simulink model "VTOL_6D0F_control"  (R2023a)
settings: Solver=VariableStepAuto  StartTime=0.0  StopTime=100  RelTol=1e-3
values from neighbouring files (symbols this model uses):
  A_lat = [Y_beta/u0  Y_p/u0  -(1-(Y_r)/(u0))  g/u0 ; L_beta  L_p  L_r  0  ;N_beta  N_p N_r 0  ; 0 1 0 0 ]    [vtol_script.m]
  A_long = [Xu Xw   0  -g  0; Zu Zw  u0 0  0 ; Mu+Mwdot*Zu  Mw+Mwdot*Zw  Mq+Mwdot*u0  0  0; 0  0  1  0  0 ; 0 0 0 k0  0]    [vtol_script.m]
  B_lat = [0 Y_delr/u0 ; L_dela   L_delr; N_dela N_delr ; 0 0]    [vtol_script.m]
  B_long = [ Xd XdT ; Zde   ZdT; Md  MdT; 0 0 ;0 0]    [vtol_script.m]
  C_lat = eye(4)    [vtol_script.m]
  C_long = eye(5)    [vtol_script.m]
  C_p = K_T/(0.5*rho*S_p*(R_p)^2)    (= 0.0365795108738)    [vtol_script.m]
  D_lat = zeros(4,2)    [vtol_script.m]
  D_long = [ 0 0; 0 0; 0 0; 0 0; 0 0]    [vtol_script.m]
  guidance_mode_on = 1    [vtol_script.m]
  K_motor = 942.3726    [vtol_script.m]
  q_motor = 283    [vtol_script.m]
  R_p = 0.3556/2    (= 0.1778)    [vtol_script.m]
  S_p = pi*(R_p)^2    (= 0.0993146659031)    [vtol_script.m]
  u0 = 16    [vtol_script.m]
libraries: simulink_extras x26, slpidlib x6, aerolibatmos2 x1
settings Model: Creator=manup  LastModifiedBy=manup

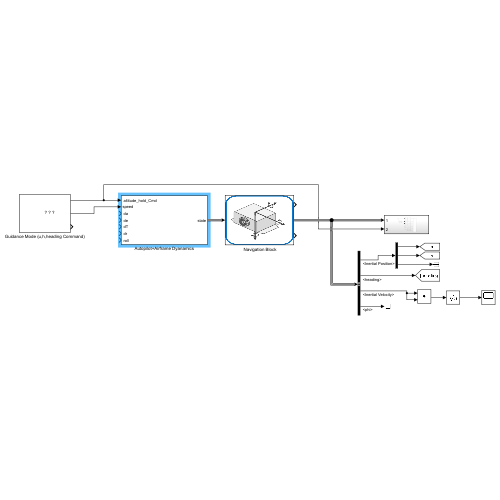
[thumbnail: Simulink's stored preview of the top-level diagram]
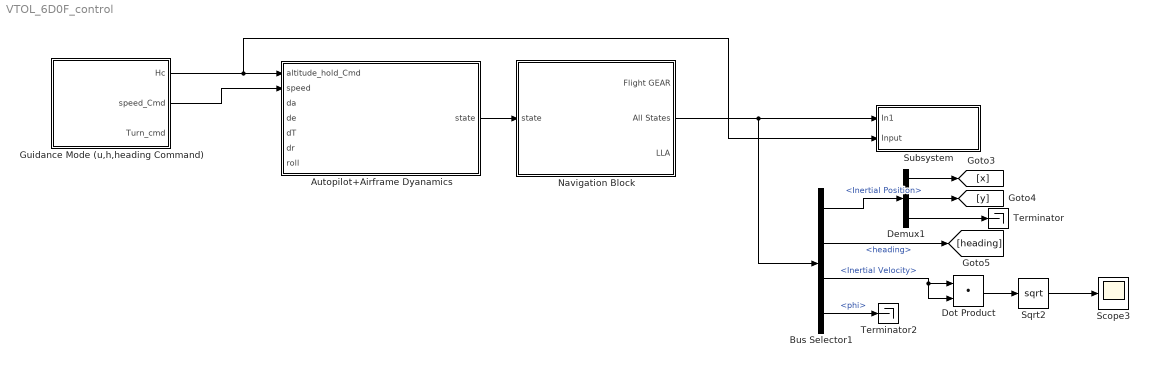
== system VTOL_6D0F_control ==
  " Navigation Block" : Subsystem
      mask Display: image('sensor.png'); % Use "Edit Image" on toolstrip to change.
  Autopilot+Airframe Dyanamics : Subsystem
  Bus Selector1 : BusSelector  OutputSignals=Inertial Position,heading,Inertial Velocity,states.phi
  Demux1 : Demux  Outputs=03
  Dot Product : DotProduct  OutDataTypeStr=Inherit: Inherit via internal rule
  Guidance Mode (u,h,heading Command) : Subsystem
      mask Display: image('guidance.jpg'); % Use "Edit Image" on toolstrip to change.
  Scope3 : Scope
  Sqrt2 : Sqrt
  Subsystem : Subsystem
  Terminator : Terminator
  Terminator2 : Terminator
  wires:
  " Navigation Block"/2(" All States") -> Bus Selector1/1, Subsystem/1(In1)
  Demux1/1 -> [x]
  Bus Selector1/4 -> Terminator2/1  "<phi>"
  Autopilot+Airframe Dyanamics/1(" state") -> " Navigation Block"/1(" state")
  Demux1/3 -> Terminator/1
  Demux1/2 -> [y]
  Bus Selector1/2 -> [heading]  "<heading>"
  Bus Selector1/3 -> Dot Product/2, Dot Product/1  "<Inertial Velocity>"
  Guidance Mode (u,h,heading Command)/1(Hc) -> Autopilot+Airframe Dyanamics/1(" altitude_hold_Cmd"), Subsystem/2(Input)
  Dot Product/1 -> Sqrt2/1
  Guidance Mode (u,h,heading Command)/2(speed_Cmd) -> Autopilot+Airframe Dyanamics/2(speed)
  Bus Selector1/1 -> Demux1/1  "<Inertial Position>"
  Sqrt2/1 -> Scope3/1

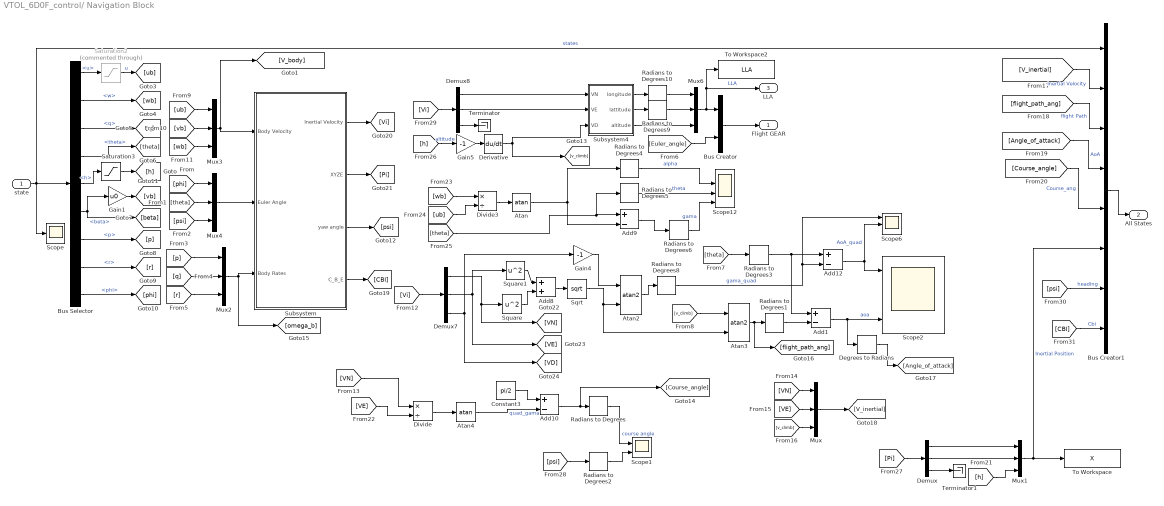
== system VTOL_6D0F_control/ Navigation Block ==
  " state" : Inport
  Add{1,9..10,12} (4 alike) : Sum  Inputs=+-
  Add8 : Sum
  Atan : Trigonometry  Operator=atan
  Atan2 : Trigonometry  Operator=atan2
  Atan3 : Trigonometry  Operator=atan2
  Atan4 : Trigonometry  Operator=atan
  Bus Creator : BusCreator  Inputs=2
  Bus Creator1 : BusCreator  Inputs=8
  Bus Selector : BusSelector  OutputSignals=u,w,q,theta,h,beta,p,r,phi
  Constant3 : Constant  Value=pi/2
  Degrees to Radians : simulink_extras/Transformations/Degrees to Radians
  Demux : Demux  Outputs=03
  Demux7 : Demux  Outputs=03
  Demux8 : Demux  Outputs=03
  Derivative : Derivative
  Divide : Product  Inputs=*/
  Divide3 : Product  Inputs=*/
  Gain1 : Gain  Gain=u0
  Gain4 : Gain  Gain=-1
  Gain5 : Gain  Gain=-1
  Mux{,1..4,6} (6 alike) : Mux  Inputs=03
  Radians to Degrees{,1..6,8..10} (10 alike) : simulink_extras/Transformations/Radians to Degrees
  Saturation2 : Saturate  Commented=through  UpperLimit=20  LowerLimit=0
  Saturation3 : Saturate  UpperLimit=0  LowerLimit=-6000
  Scope : Scope
  Scope1 : Scope  NumInputPorts=2
  Scope12 : Scope  NumInputPorts=4
  Scope2 : Scope  NumInputPorts=3
  Scope6 : Scope  NumInputPorts=3
  Sqrt : Sqrt
  Square : Math  Operator=square
  Square1 : Math  Operator=square
  Subsystem : Subsystem
  Subsystem4 : Subsystem
  Terminator : Terminator
  Terminator1 : Terminator
  To Workspace : ToWorkspace  VariableName=X  SampleTime=-1
  To Workspace2 : ToWorkspace  VariableName=LLA  SampleTime=-1
  " Flight GEAR" : Outport
  " All States" : Outport  Port=2
  LLA : Outport  Port=3
  wires:
  " state"/1 -> Bus Creator1/1, Bus Selector/1, Scope/1  "states"
  Saturation3/1 -> [h]
  Gain1/1 -> [vb]
  Saturation2/1 -> [ub]  "u"
  Bus Selector/1 -> Saturation2/1  "<u>"
  Bus Selector/3 -> [q]  "<q>"
  Bus Selector/6 -> Gain1/1, [beta]  "<beta>"
  Bus Selector/8 -> [r]  "<r>"
  Bus Selector/4 -> [theta]  "<theta>"
  Bus Selector/5 -> Saturation3/1  "<h>"
  Bus Selector/9 -> [phi]  "<phi>"
  Bus Selector/7 -> [p]  "<p>"
  Bus Selector/2 -> [wb]  "<w>"
  Radians to Degrees4/1 -> Scope12/2  "alpha"
  Demux7/1 -> [VN], Square/1
  Radians to Degrees6/1 -> Scope12/4  "gama"
  Demux7/3 -> [VD], Gain4/1
  [wb] -> Divide3/1
  Gain4/1 -> Atan2/1
  Add12/1 -> Scope2/1, Scope6/2  "AoA_quad"
  [theta] -> Add9/1, Radians to Degrees5/1
  [ub] -> Divide3/2
  [h] -> Gain5/1  "altitude"
  Atan4/1 -> Add10/2  "quad_gama"
  Add10/1 -> [Course_angle], Radians to Degrees/1
  Gain5/1 -> Derivative/1
  Atan2/1 -> Radians to Degrees8/1
  Add8/1 -> Sqrt/1
  [Vi] -> Demux7/1
  Radians to Degrees5/1 -> Scope12/3  "theta"
  Divide3/1 -> Atan/1
  Constant3/1 -> Add10/1
  Add9/1 -> Radians to Degrees6/1
  Atan/1 -> Radians to Degrees4/1, Add9/2
  Square/1 -> Add8/2
  Square1/1 -> Add8/1
  Radians to Degrees8/1 -> Scope6/1, Add12/2  "gama_quad"
  [VN] -> Divide/1
  Demux7/2 -> [VE], Square1/1
  [VE] -> Divide/2
  Subsystem/1(" Inertial Velocity ") -> [Vi]
  Subsystem/2(XYZE) -> [Pi]
  Radians to Degrees/1 -> Scope1/1  "course angle"
  [ub] -> Mux3/1
  [vb] -> Mux3/2
  [wb] -> Mux3/3
  Mux3/1 -> [V_body], Subsystem/1(" Body Velocity")
  Mux6/1 -> LLA/1, To Workspace2/1, Bus Creator/1  "LLA"
  Radians to Degrees10/1 -> Mux6/1
  [Vi] -> Demux8/1
  Radians to Degrees9/1 -> Mux6/2
  Demux8/1 -> Subsystem4/1(" VN")
  Subsystem4/2(" lattitude") -> Radians to Degrees9/1
  Subsystem4/3(" altitude") -> Mux6/3
  Subsystem4/1(longitude) -> Radians to Degrees10/1
  Demux8/2 -> Subsystem4/2(" VE")
  Bus Creator/1 -> " Flight GEAR"/1
  Sqrt/1 -> Atan2/2, Atan3/2
  Derivative/1 -> Subsystem4/3(VD), [v_climb]
  Atan3/1 -> [flight_path_ang], Radians to Degrees1/1
  Radians to Degrees1/1 -> Add1/2
  Add1/1 -> Scope2/3, Degrees to Radians/1  "aoa"
  Mux4/1 -> Subsystem/2(" Euler Angle ")
  [phi] -> Mux4/1
  [theta] -> Mux4/2
  [psi] -> Mux4/3
  [p] -> Mux2/1
  [q] -> Mux2/2
  [r] -> Mux2/3
  Mux2/1 -> [omega_b], Subsystem/3(Body Rates)
  Demux8/3 -> Terminator/1
  Subsystem/3(yaw angle) -> [psi]
  [Euler_angle] -> Bus Creator/2
  [theta] -> Radians to Degrees3/1
  [v_climb] -> Atan3/1
  [VN] -> Mux/1
  [VE] -> Mux/2
  [v_climb] -> Mux/3
  Mux/1 -> [V_inertial]
  Bus Creator1/1 -> " All States"/1
  [V_inertial] -> Bus Creator1/2  "Inertial Velocity"
  [flight_path_ang] -> Bus Creator1/3  "flight Path"
  [Angle_of_attack] -> Bus Creator1/4  "AoA"
  [Course_angle] -> Bus Creator1/5  "Course_ang"
  Mux1/1 -> To Workspace/1, Bus Creator1/6  "Inertial Position"
  [h] -> Mux1/3
  [Pi] -> Demux/1
  Demux/1 -> Mux1/1
  Demux/2 -> Mux1/2
  Demux/3 -> Terminator1/1
  [psi] -> Radians to Degrees2/1
  Divide/1 -> Atan4/1
  Radians to Degrees2/1 -> Scope1/2
  [psi] -> Bus Creator1/7  "heading"
  Radians to Degrees3/1 -> Add1/1, Add12/1
  Degrees to Radians/1 -> [Angle_of_attack]
  Subsystem/4(C_B_E) -> [CBI]
  [CBI] -> Bus Creator1/8  "Cbi"

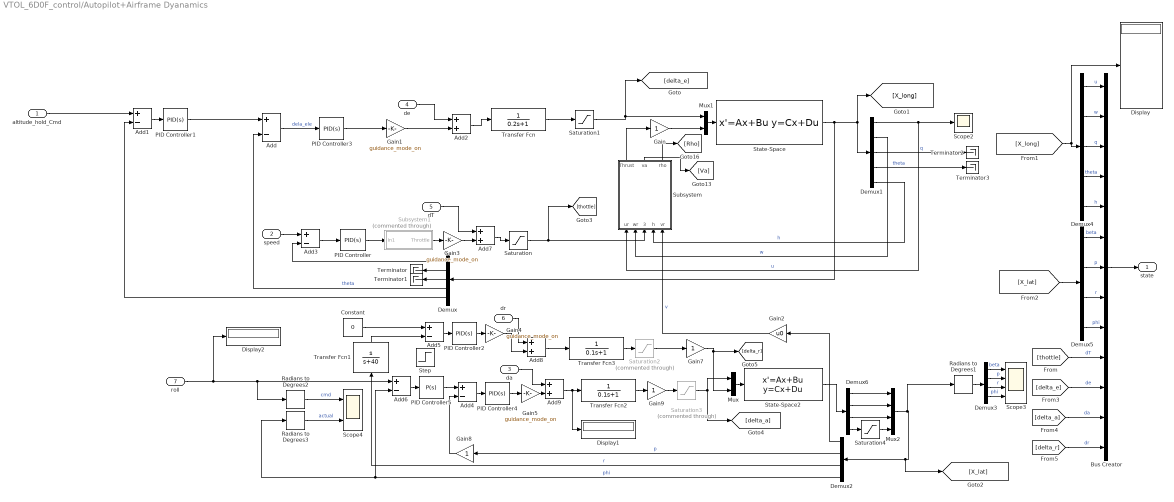
== system VTOL_6D0F_control/Autopilot+Airframe Dyanamics ==
  " altitude_hold_Cmd" : Inport
  speed : Inport  Port=2
  " da" : Inport  Port=3
  " de" : Inport  Port=4
  " dT" : Inport  Port=5
  " dr" : Inport  Port=6
  " roll" : Inport  Port=7
  Add{,1,3..6} (6 alike) : Sum  Inputs=+-
  Add{2,7..9} (4 alike) : Sum
  Bus Creator : BusCreator  Inputs=13
  Constant : Constant  Value=0
  Demux : Demux  Outputs=05
  Demux1 : Demux  Outputs=05
  Demux{2..3,5..6} (4 alike) : Demux  Outputs=04
  Demux4 : Demux  Outputs=05
  Display : Display
  Display1 : Display
  Display2 : Display
  Gain : Gain
  Gain{1,3..5} (4 alike) : Gain  Gain=guidance_mode_on
  Gain2 : Gain  Gain=u0
  Gain7 : Gain
  Gain8 : Gain  Gain=1
  Gain9 : Gain
  Mux : Mux  Inputs=2
  Mux1 : Mux  Inputs=2
  Mux2 : Mux  Inputs=04
  PID Controller : slpidlib/PID Controller  Controller=PID  Form=Parallel  TimeDomain=Continuous-time  UseExternalTs=off  SampleTime=-1  IntegratorMethod=Forward Euler  FilterMethod=Forward Euler  ControllerParametersSource=internal  P=2289.48575834425  I=747.437446989408  UseKiTs=off  D=-902.083389576885  N=0.350006005216069  UseFilter=on  TunerSelectOption=Transfer Function Based (PID Tuner App)  InitialConditionSource=internal  InitialConditionForIntegrator=0  InitialConditionForFilter=0  DifferentiatorICPrevScaledInput=0  ExternalReset=none  TrackingMode=off  Kt=1  LimitOutput=off  SatLimitsSource=internal  UpperSaturationLimit=inf  LowerSaturationLimit=-inf  LinearizeAsGain=on  AntiWindupMode=none  Kb=1  LimitIntegrator=off  UpperIntegratorSaturationLimit=inf  LowerIntegratorSaturationLimit=-inf  POutMin=[]  POutMax=[]  IOutMin=[]  IOutMax=[]  DOutMin=[]  DOutMax=[]  NOutMin=[]  NOutMax=[]  SumOutMin=[]  SumOutMax=[]  SaturationOutMin=[]  SaturationOutMax=[]  PParamMin=[]  PParamMax=[]  IParamMin=[]  IParamMax=[]  DParamMin=[]  DParamMax=[]  NParamMin=[]  NParamMax=[]  KbParamMin=[]  KbParamMax=[]  KtParamMin=[]  KtParamMax=[]  KbOutMin=[]  KbOutMax=[]  KtOutMin=[]  KtOutMax=[]  IntegratorOutMin=[]  IntegratorOutMax=[]  FilterOutMin=[]  FilterOutMax=[]  SumI1OutMin=[]  SumI1OutMax=[]  SumI2OutMin=[]  SumI2OutMax=[]  SumI3OutMin=[]  SumI3OutMax=[]  SumI4OutMin=[]  SumI4OutMax=[]  SumDOutMin=[]  SumDOutMax=[]  DifferentiatorOutMin=[]  DifferentiatorOutMax=[]  FilterDiffOutCoefMin=[]  FilterDiffOutCoefMax=[]  ReciprocalOutMin=[]  ReciprocalOutMax=[]  SumDenOutMin=[]  SumDenOutMax=[]  SumNumOutMin=[]  SumNumOutMax=[]  DivideOutMin=[]  DivideOutMax=[]  UdiffTsProdOutMin=[]  UdiffTsProdOutMax=[]  NTsProdOutMin=[]  NTsProdOutMax=[]  UintegralTsProdOutMin=[]  UintegralTsProdOutMax=[]  UngainTsProdOutMin=[]  UngainTsProdOutMax=[]  ClampingZeroOutDataTypeStr=Inherit: Inherit via back propagation  ClampingZeroOutMin=[]  ClampingZeroOutMax=[]  FilterDenConstantOutDataTypeStr=Inherit: Inherit via back propagation  FilterDenConstantOutMin=[]  FilterDenConstantOutMax=[]  PCopyOutDataTypeStr=Inherit: Inherit via back propagation  PCopyOutMin=[]  PCopyOutMax=[]  NCopyOutDataTypeStr=Inherit: Inherit via back propagation  NCopyOutMin=[]  NCopyOutMax=[]  IntegratorContinuousStateAttributes=''  IntegratorStateMustResolveToSignalObject=off  IntegratorRTWStateStorageClass=Auto  FilterContinuousStateAttributes=''  FilterStateMustResolveToSignalObject=off  FilterRTWStateStorageClass=Auto  ParallelPVariant=InternalParameters  IdealPVariant=Disabled  IVariant=InternalParameters  DVariant=InternalParameters  IntegratorVariant=Continuous  SatVariant=Disabled  AWVariant=Passthrough  PCopyVariant=Disabled  TRVariant=Disabled  FdbkBlocksVariant=Forward  IdealPFdbkVariant=Disabled  SatFdbkVariant=Disabled  DerivativeFilterVariant=ContFilter  NVariant=InternalParameters  NCopyVariant=Disabled  FilterICVariant=InternalICsFilter  IntegratorICVariant=InternalICs  ExternalResetVariant=Disabled  TRSumVariant=Passthrough  SumFdbkVariant=Disabled  SumVariant=Sum_PID  TsampFilterVariant=InternalTs  TsampNgainVariant=Passthrough  TsampIntegralVariant=Disabled_SignalSpec  ExternalSaturationOutDataTypeStr=Inherit: Same as second input
  PID Controller1 : slpidlib/PID Controller  Controller=PID  Form=Parallel  TimeDomain=Continuous-time  UseExternalTs=off  SampleTime=-1  IntegratorMethod=Forward Euler  FilterMethod=Forward Euler  ControllerParametersSource=internal  P=-0.00607559609713456  I=-7.12616824701196e-05  UseKiTs=off  D=-0.104565196845911  N=0.496463634396692  UseFilter=on  TunerSelectOption=Transfer Function Based (PID Tuner App)  InitialConditionSource=internal  InitialConditionForIntegrator=0  InitialConditionForFilter=0  DifferentiatorICPrevScaledInput=0  ExternalReset=none  TrackingMode=off  Kt=1  LimitOutput=off  SatLimitsSource=internal  UpperSaturationLimit=inf  LowerSaturationLimit=-inf  LinearizeAsGain=on  AntiWindupMode=none  Kb=1  LimitIntegrator=off  UpperIntegratorSaturationLimit=inf  LowerIntegratorSaturationLimit=-inf  POutMin=[]  POutMax=[]  IOutMin=[]  IOutMax=[]  DOutMin=[]  DOutMax=[]  NOutMin=[]  NOutMax=[]  SumOutMin=[]  SumOutMax=[]  SaturationOutMin=[]  SaturationOutMax=[]  PParamMin=[]  PParamMax=[]  IParamMin=[]  IParamMax=[]  DParamMin=[]  DParamMax=[]  NParamMin=[]  NParamMax=[]  KbParamMin=[]  KbParamMax=[]  KtParamMin=[]  KtParamMax=[]  KbOutMin=[]  KbOutMax=[]  KtOutMin=[]  KtOutMax=[]  IntegratorOutMin=[]  IntegratorOutMax=[]  FilterOutMin=[]  FilterOutMax=[]  SumI1OutMin=[]  SumI1OutMax=[]  SumI2OutMin=[]  SumI2OutMax=[]  SumI3OutMin=[]  SumI3OutMax=[]  SumI4OutMin=[]  SumI4OutMax=[]  SumDOutMin=[]  SumDOutMax=[]  DifferentiatorOutMin=[]  DifferentiatorOutMax=[]  FilterDiffOutCoefMin=[]  FilterDiffOutCoefMax=[]  ReciprocalOutMin=[]  ReciprocalOutMax=[]  SumDenOutMin=[]  SumDenOutMax=[]  SumNumOutMin=[]  SumNumOutMax=[]  DivideOutMin=[]  DivideOutMax=[]  UdiffTsProdOutMin=[]  UdiffTsProdOutMax=[]  NTsProdOutMin=[]  NTsProdOutMax=[]  UintegralTsProdOutMin=[]  UintegralTsProdOutMax=[]  UngainTsProdOutMin=[]  UngainTsProdOutMax=[]  ClampingZeroOutDataTypeStr=Inherit: Inherit via back propagation  ClampingZeroOutMin=[]  ClampingZeroOutMax=[]  FilterDenConstantOutDataTypeStr=Inherit: Inherit via back propagation  FilterDenConstantOutMin=[]  FilterDenConstantOutMax=[]  PCopyOutDataTypeStr=Inherit: Inherit via back propagation  PCopyOutMin=[]  PCopyOutMax=[]  NCopyOutDataTypeStr=Inherit: Inherit via back propagation  NCopyOutMin=[]  NCopyOutMax=[]  IntegratorContinuousStateAttributes=''  IntegratorStateMustResolveToSignalObject=off  IntegratorRTWStateStorageClass=Auto  FilterContinuousStateAttributes=''  FilterStateMustResolveToSignalObject=off  FilterRTWStateStorageClass=Auto  ParallelPVariant=InternalParameters  IdealPVariant=Disabled  IVariant=InternalParameters  DVariant=InternalParameters  IntegratorVariant=Continuous  SatVariant=Disabled  AWVariant=Passthrough  PCopyVariant=Disabled  TRVariant=Disabled  FdbkBlocksVariant=Forward  IdealPFdbkVariant=Disabled  SatFdbkVariant=Disabled  DerivativeFilterVariant=ContFilter  NVariant=InternalParameters  NCopyVariant=Disabled  FilterICVariant=InternalICsFilter  IntegratorICVariant=InternalICs  ExternalResetVariant=Disabled  TRSumVariant=Passthrough  SumFdbkVariant=Disabled  SumVariant=Sum_PID  TsampFilterVariant=InternalTs  TsampNgainVariant=Passthrough  TsampIntegralVariant=Disabled_SignalSpec  ExternalSaturationOutDataTypeStr=Inherit: Same as second input
  PID Controller2 : slpidlib/PID Controller  Controller=PID  Form=Parallel  TimeDomain=Continuous-time  UseExternalTs=off  SampleTime=-1  IntegratorMethod=Forward Euler  FilterMethod=Forward Euler  ControllerParametersSource=internal  P=1.24983649640651  I=1.358016248583  UseKiTs=off  D=-6.073149463355  N=0.205797091599334  UseFilter=on  TunerSelectOption=Transfer Function Based (PID Tuner App)  InitialConditionSource=internal  InitialConditionForIntegrator=0  InitialConditionForFilter=0  DifferentiatorICPrevScaledInput=0  ExternalReset=none  TrackingMode=off  Kt=1  LimitOutput=off  SatLimitsSource=internal  UpperSaturationLimit=inf  LowerSaturationLimit=-inf  LinearizeAsGain=on  AntiWindupMode=none  Kb=1  LimitIntegrator=off  UpperIntegratorSaturationLimit=inf  LowerIntegratorSaturationLimit=-inf  POutMin=[]  POutMax=[]  IOutMin=[]  IOutMax=[]  DOutMin=[]  DOutMax=[]  NOutMin=[]  NOutMax=[]  SumOutMin=[]  SumOutMax=[]  SaturationOutMin=[]  SaturationOutMax=[]  PParamMin=[]  PParamMax=[]  IParamMin=[]  IParamMax=[]  DParamMin=[]  DParamMax=[]  NParamMin=[]  NParamMax=[]  KbParamMin=[]  KbParamMax=[]  KtParamMin=[]  KtParamMax=[]  KbOutMin=[]  KbOutMax=[]  KtOutMin=[]  KtOutMax=[]  IntegratorOutMin=[]  IntegratorOutMax=[]  FilterOutMin=[]  FilterOutMax=[]  SumI1OutMin=[]  SumI1OutMax=[]  SumI2OutMin=[]  SumI2OutMax=[]  SumI3OutMin=[]  SumI3OutMax=[]  SumI4OutMin=[]  SumI4OutMax=[]  SumDOutMin=[]  SumDOutMax=[]  DifferentiatorOutMin=[]  DifferentiatorOutMax=[]  FilterDiffOutCoefMin=[]  FilterDiffOutCoefMax=[]  ReciprocalOutMin=[]  ReciprocalOutMax=[]  SumDenOutMin=[]  SumDenOutMax=[]  SumNumOutMin=[]  SumNumOutMax=[]  DivideOutMin=[]  DivideOutMax=[]  UdiffTsProdOutMin=[]  UdiffTsProdOutMax=[]  NTsProdOutMin=[]  NTsProdOutMax=[]  UintegralTsProdOutMin=[]  UintegralTsProdOutMax=[]  UngainTsProdOutMin=[]  UngainTsProdOutMax=[]  ClampingZeroOutDataTypeStr=Inherit: Inherit via back propagation  ClampingZeroOutMin=[]  ClampingZeroOutMax=[]  FilterDenConstantOutDataTypeStr=Inherit: Inherit via back propagation  FilterDenConstantOutMin=[]  FilterDenConstantOutMax=[]  PCopyOutDataTypeStr=Inherit: Inherit via back propagation  PCopyOutMin=[]  PCopyOutMax=[]  NCopyOutDataTypeStr=Inherit: Inherit via back propagation  NCopyOutMin=[]  NCopyOutMax=[]  IntegratorContinuousStateAttributes=''  IntegratorStateMustResolveToSignalObject=off  IntegratorRTWStateStorageClass=Auto  FilterContinuousStateAttributes=''  FilterStateMustResolveToSignalObject=off  FilterRTWStateStorageClass=Auto  ParallelPVariant=InternalParameters  IdealPVariant=Disabled  IVariant=InternalParameters  DVariant=InternalParameters  IntegratorVariant=Continuous  SatVariant=Disabled  AWVariant=Passthrough  PCopyVariant=Disabled  TRVariant=Disabled  FdbkBlocksVariant=Forward  IdealPFdbkVariant=Disabled  SatFdbkVariant=Disabled  DerivativeFilterVariant=ContFilter  NVariant=InternalParameters  NCopyVariant=Disabled  FilterICVariant=InternalICsFilter  IntegratorICVariant=InternalICs  ExternalResetVariant=Disabled  TRSumVariant=Passthrough  SumFdbkVariant=Disabled  SumVariant=Sum_PID  TsampFilterVariant=InternalTs  TsampNgainVariant=Passthrough  TsampIntegralVariant=Disabled_SignalSpec  ExternalSaturationOutDataTypeStr=Inherit: Same as second input
  PID Controller3 : slpidlib/PID Controller  Controller=PID  Form=Parallel  TimeDomain=Continuous-time  UseExternalTs=off  SampleTime=-1  IntegratorMethod=Forward Euler  FilterMethod=Forward Euler  ControllerParametersSource=internal  P=-0.0213069977558539  I=-0.000289283901321069  UseKiTs=off  D=0.00377457345522127  N=5.64487564187695  UseFilter=on  TunerSelectOption=Transfer Function Based (PID Tuner App)  InitialConditionSource=internal  InitialConditionForIntegrator=0  InitialConditionForFilter=0  DifferentiatorICPrevScaledInput=0  ExternalReset=none  TrackingMode=off  Kt=1  LimitOutput=off  SatLimitsSource=internal  UpperSaturationLimit=inf  LowerSaturationLimit=-inf  LinearizeAsGain=on  AntiWindupMode=none  Kb=1  LimitIntegrator=off  UpperIntegratorSaturationLimit=inf  LowerIntegratorSaturationLimit=-inf  POutMin=[]  POutMax=[]  IOutMin=[]  IOutMax=[]  DOutMin=[]  DOutMax=[]  NOutMin=[]  NOutMax=[]  SumOutMin=[]  SumOutMax=[]  SaturationOutMin=[]  SaturationOutMax=[]  PParamMin=[]  PParamMax=[]  IParamMin=[]  IParamMax=[]  DParamMin=[]  DParamMax=[]  NParamMin=[]  NParamMax=[]  KbParamMin=[]  KbParamMax=[]  KtParamMin=[]  KtParamMax=[]  KbOutMin=[]  KbOutMax=[]  KtOutMin=[]  KtOutMax=[]  IntegratorOutMin=[]  IntegratorOutMax=[]  FilterOutMin=[]  FilterOutMax=[]  SumI1OutMin=[]  SumI1OutMax=[]  SumI2OutMin=[]  SumI2OutMax=[]  SumI3OutMin=[]  SumI3OutMax=[]  SumI4OutMin=[]  SumI4OutMax=[]  SumDOutMin=[]  SumDOutMax=[]  DifferentiatorOutMin=[]  DifferentiatorOutMax=[]  FilterDiffOutCoefMin=[]  FilterDiffOutCoefMax=[]  ReciprocalOutMin=[]  ReciprocalOutMax=[]  SumDenOutMin=[]  SumDenOutMax=[]  SumNumOutMin=[]  SumNumOutMax=[]  DivideOutMin=[]  DivideOutMax=[]  UdiffTsProdOutMin=[]  UdiffTsProdOutMax=[]  NTsProdOutMin=[]  NTsProdOutMax=[]  UintegralTsProdOutMin=[]  UintegralTsProdOutMax=[]  UngainTsProdOutMin=[]  UngainTsProdOutMax=[]  ClampingZeroOutDataTypeStr=Inherit: Inherit via back propagation  ClampingZeroOutMin=[]  ClampingZeroOutMax=[]  FilterDenConstantOutDataTypeStr=Inherit: Inherit via back propagation  FilterDenConstantOutMin=[]  FilterDenConstantOutMax=[]  PCopyOutDataTypeStr=Inherit: Inherit via back propagation  PCopyOutMin=[]  PCopyOutMax=[]  NCopyOutDataTypeStr=Inherit: Inherit via back propagation  NCopyOutMin=[]  NCopyOutMax=[]  IntegratorContinuousStateAttributes=''  IntegratorStateMustResolveToSignalObject=off  IntegratorRTWStateStorageClass=Auto  FilterContinuousStateAttributes=''  FilterStateMustResolveToSignalObject=off  FilterRTWStateStorageClass=Auto  ParallelPVariant=InternalParameters  IdealPVariant=Disabled  IVariant=InternalParameters  DVariant=InternalParameters  IntegratorVariant=Continuous  SatVariant=Disabled  AWVariant=Passthrough  PCopyVariant=Disabled  TRVariant=Disabled  FdbkBlocksVariant=Forward  IdealPFdbkVariant=Disabled  SatFdbkVariant=Disabled  DerivativeFilterVariant=ContFilter  NVariant=InternalParameters  NCopyVariant=Disabled  FilterICVariant=InternalICsFilter  IntegratorICVariant=InternalICs  ExternalResetVariant=Disabled  TRSumVariant=Passthrough  SumFdbkVariant=Disabled  SumVariant=Sum_PID  TsampFilterVariant=InternalTs  TsampNgainVariant=Passthrough  TsampIntegralVariant=Disabled_SignalSpec  ExternalSaturationOutDataTypeStr=Inherit: Same as second input
  PID Controller4 : slpidlib/PID Controller  Controller=PID  Form=Parallel  TimeDomain=Continuous-time  UseExternalTs=off  SampleTime=-1  IntegratorMethod=Forward Euler  FilterMethod=Forward Euler  ControllerParametersSource=internal  P=0.08122  I=1.4278  UseKiTs=off  D=0.0046499  N=100  UseFilter=on  TunerSelectOption=Transfer Function Based (PID Tuner App)  InitialConditionSource=internal  InitialConditionForIntegrator=0  InitialConditionForFilter=0  DifferentiatorICPrevScaledInput=0  ExternalReset=none  TrackingMode=off  Kt=1  LimitOutput=off  SatLimitsSource=internal  UpperSaturationLimit=inf  LowerSaturationLimit=-inf  LinearizeAsGain=on  AntiWindupMode=none  Kb=1  LimitIntegrator=off  UpperIntegratorSaturationLimit=inf  LowerIntegratorSaturationLimit=-inf  POutMin=[]  POutMax=[]  IOutMin=[]  IOutMax=[]  DOutMin=[]  DOutMax=[]  NOutMin=[]  NOutMax=[]  SumOutMin=[]  SumOutMax=[]  SaturationOutMin=[]  SaturationOutMax=[]  PParamMin=[]  PParamMax=[]  IParamMin=[]  IParamMax=[]  DParamMin=[]  DParamMax=[]  NParamMin=[]  NParamMax=[]  KbParamMin=[]  KbParamMax=[]  KtParamMin=[]  KtParamMax=[]  KbOutMin=[]  KbOutMax=[]  KtOutMin=[]  KtOutMax=[]  IntegratorOutMin=[]  IntegratorOutMax=[]  FilterOutMin=[]  FilterOutMax=[]  SumI1OutMin=[]  SumI1OutMax=[]  SumI2OutMin=[]  SumI2OutMax=[]  SumI3OutMin=[]  SumI3OutMax=[]  SumI4OutMin=[]  SumI4OutMax=[]  SumDOutMin=[]  SumDOutMax=[]  DifferentiatorOutMin=[]  DifferentiatorOutMax=[]  FilterDiffOutCoefMin=[]  FilterDiffOutCoefMax=[]  ReciprocalOutMin=[]  ReciprocalOutMax=[]  SumDenOutMin=[]  SumDenOutMax=[]  SumNumOutMin=[]  SumNumOutMax=[]  DivideOutMin=[]  DivideOutMax=[]  UdiffTsProdOutMin=[]  UdiffTsProdOutMax=[]  NTsProdOutMin=[]  NTsProdOutMax=[]  UintegralTsProdOutMin=[]  UintegralTsProdOutMax=[]  UngainTsProdOutMin=[]  UngainTsProdOutMax=[]  ClampingZeroOutDataTypeStr=Inherit: Inherit via back propagation  ClampingZeroOutMin=[]  ClampingZeroOutMax=[]  FilterDenConstantOutDataTypeStr=Inherit: Inherit via back propagation  FilterDenConstantOutMin=[]  FilterDenConstantOutMax=[]  PCopyOutDataTypeStr=Inherit: Inherit via back propagation  PCopyOutMin=[]  PCopyOutMax=[]  NCopyOutDataTypeStr=Inherit: Inherit via back propagation  NCopyOutMin=[]  NCopyOutMax=[]  IntegratorContinuousStateAttributes=''  IntegratorStateMustResolveToSignalObject=off  IntegratorRTWStateStorageClass=Auto  FilterContinuousStateAttributes=''  FilterStateMustResolveToSignalObject=off  FilterRTWStateStorageClass=Auto  ParallelPVariant=InternalParameters  IdealPVariant=Disabled  IVariant=InternalParameters  DVariant=InternalParameters  IntegratorVariant=Continuous  SatVariant=Disabled  AWVariant=Passthrough  PCopyVariant=Disabled  TRVariant=Disabled  FdbkBlocksVariant=Forward  IdealPFdbkVariant=Disabled  SatFdbkVariant=Disabled  DerivativeFilterVariant=ContFilter  NVariant=InternalParameters  NCopyVariant=Disabled  FilterICVariant=InternalICsFilter  IntegratorICVariant=InternalICs  ExternalResetVariant=Disabled  TRSumVariant=Passthrough  SumFdbkVariant=Disabled  SumVariant=Sum_PID  TsampFilterVariant=InternalTs  TsampNgainVariant=Passthrough  TsampIntegralVariant=Disabled_SignalSpec  ExternalSaturationOutDataTypeStr=Inherit: Same as second input
  PID Controller5 : slpidlib/PID Controller  Controller=P  Form=Parallel  TimeDomain=Continuous-time  UseExternalTs=off  SampleTime=-1  IntegratorMethod=Forward Euler  FilterMethod=Forward Euler  ControllerParametersSource=internal  P=1.34509  I=86.5946257976551  UseKiTs=off  D=0  N=100  UseFilter=on  TunerSelectOption=Transfer Function Based (PID Tuner App)  InitialConditionSource=internal  InitialConditionForIntegrator=0  InitialConditionForFilter=0  DifferentiatorICPrevScaledInput=0  ExternalReset=none  TrackingMode=off  Kt=1  LimitOutput=off  SatLimitsSource=internal  UpperSaturationLimit=inf  LowerSaturationLimit=-inf  LinearizeAsGain=on  AntiWindupMode=none  Kb=1  LimitIntegrator=off  UpperIntegratorSaturationLimit=inf  LowerIntegratorSaturationLimit=-inf  POutMin=[]  POutMax=[]  IOutMin=[]  IOutMax=[]  DOutMin=[]  DOutMax=[]  NOutMin=[]  NOutMax=[]  SumOutMin=[]  SumOutMax=[]  SaturationOutMin=[]  SaturationOutMax=[]  PParamMin=[]  PParamMax=[]  IParamMin=[]  IParamMax=[]  DParamMin=[]  DParamMax=[]  NParamMin=[]  NParamMax=[]  KbParamMin=[]  KbParamMax=[]  KtParamMin=[]  KtParamMax=[]  KbOutMin=[]  KbOutMax=[]  KtOutMin=[]  KtOutMax=[]  IntegratorOutMin=[]  IntegratorOutMax=[]  FilterOutMin=[]  FilterOutMax=[]  SumI1OutMin=[]  SumI1OutMax=[]  SumI2OutMin=[]  SumI2OutMax=[]  SumI3OutMin=[]  SumI3OutMax=[]  SumI4OutMin=[]  SumI4OutMax=[]  SumDOutMin=[]  SumDOutMax=[]  DifferentiatorOutMin=[]  DifferentiatorOutMax=[]  FilterDiffOutCoefMin=[]  FilterDiffOutCoefMax=[]  ReciprocalOutMin=[]  ReciprocalOutMax=[]  SumDenOutMin=[]  SumDenOutMax=[]  SumNumOutMin=[]  SumNumOutMax=[]  DivideOutMin=[]  DivideOutMax=[]  UdiffTsProdOutMin=[]  UdiffTsProdOutMax=[]  NTsProdOutMin=[]  NTsProdOutMax=[]  UintegralTsProdOutMin=[]  UintegralTsProdOutMax=[]  UngainTsProdOutMin=[]  UngainTsProdOutMax=[]  ClampingZeroOutDataTypeStr=Inherit: Inherit via back propagation  ClampingZeroOutMin=[]  ClampingZeroOutMax=[]  FilterDenConstantOutDataTypeStr=Inherit: Inherit via back propagation  FilterDenConstantOutMin=[]  FilterDenConstantOutMax=[]  PCopyOutDataTypeStr=Inherit: Inherit via back propagation  PCopyOutMin=[]  PCopyOutMax=[]  NCopyOutDataTypeStr=Inherit: Inherit via back propagation  NCopyOutMin=[]  NCopyOutMax=[]  IntegratorContinuousStateAttributes=''  IntegratorStateMustResolveToSignalObject=off  IntegratorRTWStateStorageClass=Auto  FilterContinuousStateAttributes=''  FilterStateMustResolveToSignalObject=off  FilterRTWStateStorageClass=Auto  ParallelPVariant=InternalParameters  IdealPVariant=Disabled  IVariant=Disabled  DVariant=Disabled  IntegratorVariant=Disabled  SatVariant=Disabled  AWVariant=Disabled  PCopyVariant=Disabled  TRVariant=Disabled  FdbkBlocksVariant=Forward  IdealPFdbkVariant=Disabled  SatFdbkVariant=Disabled  DerivativeFilterVariant=Disabled  NVariant=Disabled  NCopyVariant=Disabled_SignalSpec  FilterICVariant=Disabled  IntegratorICVariant=Disabled  ExternalResetVariant=Disabled  TRSumVariant=Passthrough  SumFdbkVariant=Disabled  SumVariant=Passthrough_P  TsampFilterVariant=InternalTs  TsampNgainVariant=Passthrough  TsampIntegralVariant=Disabled_SignalSpec  ExternalSaturationOutDataTypeStr=Inherit: Same as second input
  Radians to Degrees1 : simulink_extras/Transformations/Radians to Degrees
  Radians to Degrees2 : simulink_extras/Transformations/Radians to Degrees
  Radians to Degrees3 : simulink_extras/Transformations/Radians to Degrees
  Saturation : Saturate  UpperLimit=100  LowerLimit=0
  Saturation1 : Saturate  UpperLimit=pi/4  LowerLimit=-pi/4
  Saturation2 : Saturate  Commented=through  UpperLimit=pi/6  LowerLimit=-pi/6
  Saturation3 : Saturate  Commented=through  UpperLimit=pi/12  LowerLimit=-pi/12
  Saturation4 : Saturate  UpperLimit=pi/4  LowerLimit=-pi/4
  Scope2 : Scope
  Scope3 : Scope  NumInputPorts=4
  Scope4 : Scope  NumInputPorts=2
  State-Space : StateSpace  A=A_long  B=B_long  C=C_long  D=D_long  InitialCondition=[5 0 0 0 0]'  ParameterTunability=Unconstrained
  State-Space2 : StateSpace  A=A_lat  B=B_lat  C=C_lat  D=D_lat  InitialCondition=0
  Step : Step  Time=0  SampleTime=0
  Subsystem : Subsystem
  Subsystem1 : Subsystem  Commented=through
  Terminator{,1..3} (4 alike) : Terminator
  Transfer Fcn : TransferFcn  Denominator="[0.2  1]"
  Transfer Fcn1 : TransferFcn  Numerator="[1  0]"  Denominator="[1  40]"
  Transfer Fcn2 : TransferFcn  Denominator="[0.1  1]"
  Transfer Fcn3 : TransferFcn  Denominator="[0.1  1]"
  " state" : Outport
  wires:
  PID Controller2/1 -> Gain4/1
  Demux1/1 -> Scope2/1, Subsystem/1(ur)  "u"
  Subsystem/3(" rho") -> [Rho]
  Mux1/1 -> State-Space/1
  Transfer Fcn1/1 -> Add5/2
  Demux2/4 -> Radians to Degrees3/1, Add6/2  "phi"
  State-Space2/1 -> Demux6/1
  Transfer Fcn/1 -> Saturation1/1
  Subsystem/1(Thrust) -> Gain/1
  Add/1 -> PID Controller3/1  "dela_ele"
  Radians to Degrees1/1 -> Demux3/1
  PID Controller/1 -> Subsystem1/1(In1)
  Add1/1 -> PID Controller1/1
  Demux2/1 -> Gain2/1
  Subsystem/2(" va") -> [Va]
  Demux2/3 -> Transfer Fcn1/1  "r"
  Demux3/4 -> Scope3/4  "phi"
  Constant/1 -> Add5/1
  Demux1/2 -> Subsystem/2(wr)  "w"
  Demux3/3 -> Scope3/3  "r"
  Saturation/1 -> [thottle], Subsystem/3(" Throttle")
  Add3/1 -> PID Controller/1
  Gain2/1 -> Subsystem/5(" vr")  "v"
  State-Space/1 -> Demux/1, [X_long], Demux1/1
  Demux3/2 -> Scope3/2  "p"
  Transfer Fcn3/1 -> Saturation2/1
  Demux1/5 -> Subsystem/4(" h")  "h"
  Add5/1 -> PID Controller2/1
  Demux/1 -> Add3/2
  Add4/1 -> PID Controller4/1
  Demux3/1 -> Scope3/1  "beta"
  Mux/1 -> State-Space2/1
  Add8/1 -> Transfer Fcn3/1
  Demux/2 -> Terminator/1
  Demux/3 -> Terminator1/1
  [X_long] -> Display/1, Demux4/1
  Demux4/1 -> Bus Creator/1  "u"
  Demux4/2 -> Bus Creator/2  "w"
  Demux4/3 -> Bus Creator/3  "q"
  Demux4/4 -> Bus Creator/4  "theta"
  Demux4/5 -> Bus Creator/5  "h"
  [X_lat] -> Demux5/1
  Demux5/1 -> Bus Creator/6  "beta"
  Demux5/2 -> Bus Creator/7  "p"
  Demux5/3 -> Bus Creator/8  "r"
  Demux5/4 -> Bus Creator/9  "phi"
  Bus Creator/1 -> " state"/1
  Demux1/3 -> Terminator2/1  "q"
  Demux1/4 -> Terminator3/1  "theta"
  Demux/5 -> Add1/2
  PID Controller3/1 -> Gain1/1
  Add2/1 -> Transfer Fcn/1
  Subsystem1/1(" Throttle") -> Gain3/1
  Add7/1 -> Saturation/1
  PID Controller4/1 -> Gain5/1
  Add9/1 -> Display1/1, Transfer Fcn2/1
  " da"/1 -> Add9/1
  " de"/1 -> Add2/1
  " dT"/1 -> Add7/1
  " dr"/1 -> Add8/1
  Gain1/1 -> Add2/2
  Gain3/1 -> Add7/2
  Gain4/1 -> Add8/2
  Gain5/1 -> Add9/2
  [thottle] -> Bus Creator/10  "dT"
  [delta_e] -> Bus Creator/11  "de"
  [delta_a] -> Bus Creator/12  "da"
  [delta_r] -> Bus Creator/13  "dr"
  speed/1 -> Add3/1
  Gain/1 -> Mux1/2
  Gain7/1 -> [delta_r], Mux/2
  Demux2/2 -> Gain8/1  "p"
  Gain8/1 -> Add4/2
  Radians to Degrees2/1 -> Scope4/1  "cmd"
  Radians to Degrees3/1 -> Scope4/2  "actual"
  Transfer Fcn2/1 -> Gain9/1
  Gain9/1 -> Saturation3/1
  Add6/1 -> PID Controller5/1
  " altitude_hold_Cmd"/1 -> Add1/1
  Saturation1/1 -> [delta_e], Mux1/1
  Saturation2/1 -> Gain7/1
  Saturation3/1 -> Mux/1, [delta_a]
  Demux6/4 -> Saturation4/1
  Demux6/1 -> Mux2/1
  Demux6/2 -> Mux2/2
  Demux6/3 -> Mux2/3
  Saturation4/1 -> Mux2/4
  Mux2/1 -> Radians to Degrees1/1, [X_lat], Demux2/1
  " roll"/1 -> Radians to Degrees2/1, Add6/1, Display2/1
  PID Controller5/1 -> Add4/1
  Demux/4 -> Add/2  "theta"
  PID Controller1/1 -> Add/1

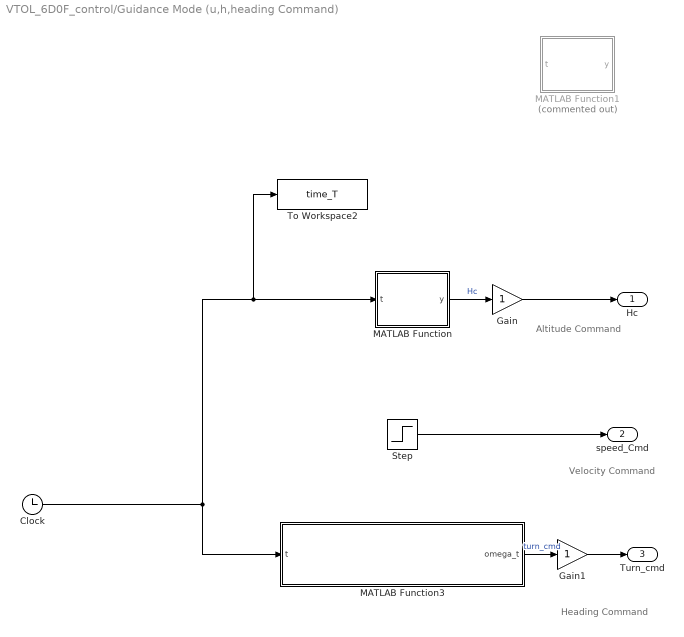
== system VTOL_6D0F_control/Guidance Mode (u,h,heading Command) ==
  note: Velocity Command
  note: Altitude Command
  note: Heading Command
  Clock : Clock
  Gain : Gain
  Gain1 : Gain  Gain=1
  MATLAB Function : MATLAB Function  TreatAsAtomicUnit=on
  MATLAB Function1 : MATLAB Function  Commented=on  TreatAsAtomicUnit=on
  MATLAB Function3 : MATLAB Function  TreatAsAtomicUnit=on
  Step : Step  Time=0  After=15  SampleTime=0
  To Workspace2 : ToWorkspace  VariableName=time_T  SampleTime=-1
  Hc : Outport
  speed_Cmd : Outport  Port=2
  Turn_cmd : Outport  Port=3
  wires:
  MATLAB Function3/1(omega_t) -> Gain1/1  "turn_cmd"
  Step/1 -> speed_Cmd/1
  MATLAB Function/1(y) -> Gain/1  "Hc"
  Clock/1 -> MATLAB Function/1(t), To Workspace2/1, MATLAB Function3/1(t)
  Gain1/1 -> Turn_cmd/1
  Gain/1 -> Hc/1

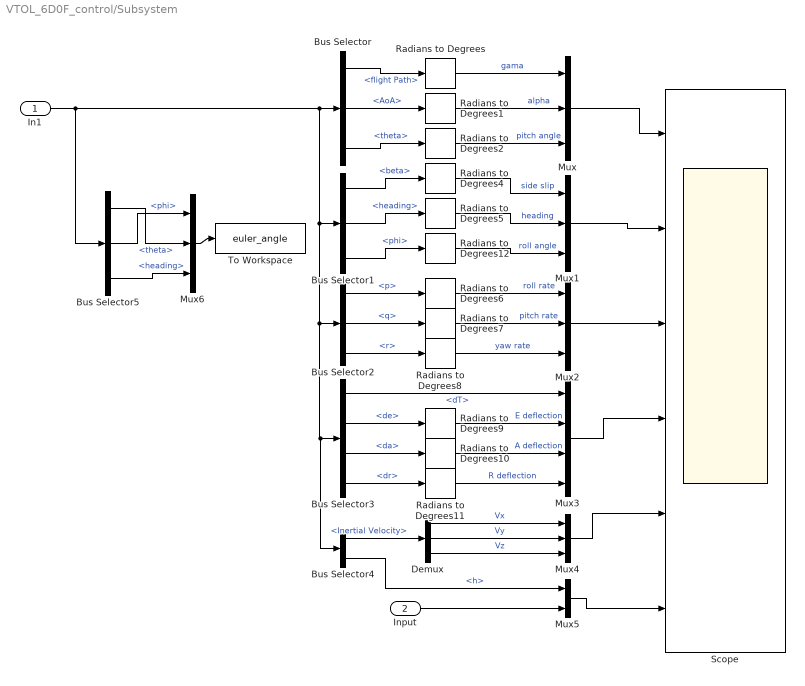
== system VTOL_6D0F_control/Subsystem ==
  In1 : Inport
  Input : Inport  Port=2
  Bus Selector : BusSelector  OutputSignals=flight Path,AoA,states.theta
  Bus Selector1 : BusSelector  OutputSignals=states.beta,heading,states.phi
  Bus Selector2 : BusSelector  OutputSignals=states.p,states.q,states.r
  Bus Selector3 : BusSelector  OutputSignals=states.dT,states.de,states.da,states.dr
  Bus Selector4 : BusSelector  OutputSignals=Inertial Velocity,states.h
  Bus Selector5 : BusSelector  OutputSignals=states.theta,states.phi,heading
  Demux : Demux  Outputs=03
  Mux{,1..2,4,6} (5 alike) : Mux  Inputs=03
  Mux3 : Mux  Inputs=04
  Mux5 : Mux  Inputs=2
  Radians to Degrees{,1..2,4..12} (12 alike) : simulink_extras/Transformations/Radians to Degrees
  Scope : Scope  NumInputPorts=6
  To Workspace : ToWorkspace  VariableName=euler_angle  SampleTime=-1
  wires:
  Bus Selector/1 -> Radians to Degrees/1  "<flight Path>"
  Bus Selector/2 -> Radians to Degrees1/1  "<AoA>"
  Bus Selector/3 -> Radians to Degrees2/1  "<theta>"
  Bus Selector1/1 -> Radians to Degrees4/1  "<beta>"
  Bus Selector1/2 -> Radians to Degrees5/1  "<heading>"
  Bus Selector2/1 -> Radians to Degrees6/1  "<p>"
  Bus Selector2/2 -> Radians to Degrees7/1  "<q>"
  Bus Selector2/3 -> Radians to Degrees8/1  "<r>"
  Bus Selector3/2 -> Radians to Degrees9/1  "<de>"
  Bus Selector3/3 -> Radians to Degrees10/1  "<da>"
  Bus Selector3/4 -> Radians to Degrees11/1  "<dr>"
  Bus Selector3/1 -> Mux3/1  "<dT>"
  Radians to Degrees/1 -> Mux/1  "gama"
  Radians to Degrees1/1 -> Mux/2  "alpha"
  Radians to Degrees2/1 -> Mux/3  "pitch angle"
  Radians to Degrees4/1 -> Mux1/1  "side slip"
  Radians to Degrees5/1 -> Mux1/2  "heading"
  Mux1/1 -> Scope/2
  Mux/1 -> Scope/1
  Mux2/1 -> Scope/3
  Radians to Degrees6/1 -> Mux2/1  "roll rate"
  Radians to Degrees7/1 -> Mux2/2  "pitch rate"
  Radians to Degrees8/1 -> Mux2/3  "yaw rate"
  Mux3/1 -> Scope/4
  Radians to Degrees9/1 -> Mux3/2  "E deflection"
  Radians to Degrees10/1 -> Mux3/3  "A deflection"
  Radians to Degrees11/1 -> Mux3/4  "R deflection"
  Bus Selector4/1 -> Demux/1  "<Inertial Velocity>"
  Bus Selector4/2 -> Mux5/1  "<h>"
  Demux/1 -> Mux4/1  "Vx"
  Demux/2 -> Mux4/2  "Vy"
  Demux/3 -> Mux4/3  "Vz"
  Input/1 -> Mux5/2
  Mux4/1 -> Scope/5
  Mux5/1 -> Scope/6
  In1/1 -> Bus Selector/1, Bus Selector4/1, Bus Selector3/1, Bus Selector2/1, Bus Selector1/1, Bus Selector5/1
  Bus Selector1/3 -> Radians to Degrees12/1  "<phi>"
  Radians to Degrees12/1 -> Mux1/3  "roll angle"
  Bus Selector5/2 -> Mux6/1  "<phi>"
  Bus Selector5/3 -> Mux6/3  "<heading>"
  Bus Selector5/1 -> Mux6/2  "<theta>"
  Mux6/1 -> To Workspace/1

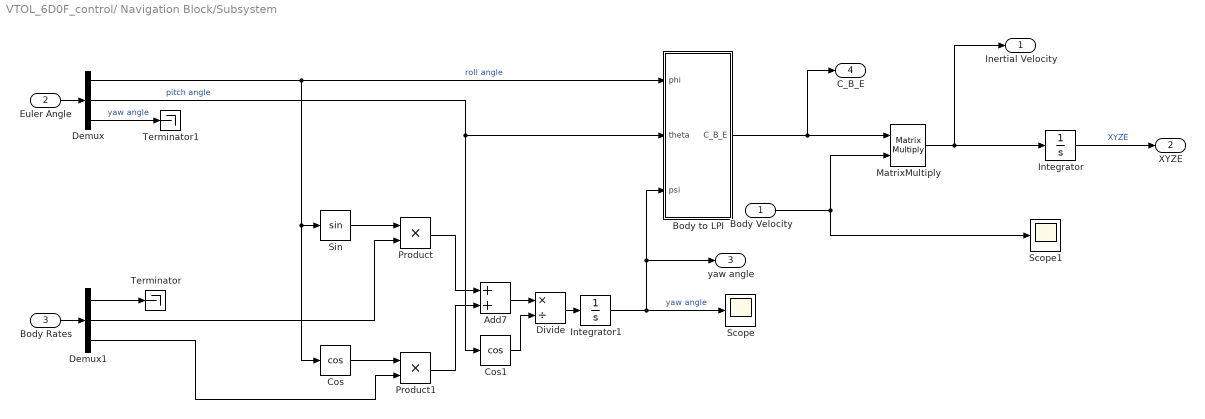
== system VTOL_6D0F_control/ Navigation Block/Subsystem ==
  " Body Velocity" : Inport
  " Euler Angle " : Inport  Port=2
  Body Rates : Inport  Port=3
  " Body to LPI" : Subsystem
  Add7 : Sum
  Cos : Trigonometry  Operator=cos
  Cos1 : Trigonometry  Operator=cos
  Demux : Demux  Outputs=03
  Demux1 : Demux  Outputs=03
  Divide : Product  Inputs=*/
  Integrator : Integrator
  Integrator1 : Integrator
  MatrixMultiply : Product  Multiplication=Matrix(*)
  Product : Product
  Product1 : Product
  Scope : Scope
  Scope1 : Scope
  Sin : Trigonometry
  Terminator : Terminator
  Terminator1 : Terminator
  " Inertial Velocity " : Outport
  XYZE : Outport  Port=2
  yaw angle : Outport  Port=3
  C_B_E : Outport  Port=4
  wires:
  Demux1/2 -> Product/2
  Integrator/1 -> XYZE/1  "XYZE"
  MatrixMultiply/1 -> Integrator/1, " Inertial Velocity "/1
  Integrator1/1 -> Scope/1, " Body to LPI"/3(psi), yaw angle/1  "yaw angle"
  Divide/1 -> Integrator1/1
  Demux/2 -> Cos1/1, " Body to LPI"/2(theta)  "pitch angle"
  Product1/1 -> Add7/2
  " Body to LPI"/1(C_B_E) -> C_B_E/1, MatrixMultiply/1
  Sin/1 -> Product/1
  Cos1/1 -> Divide/2
  Demux1/3 -> Product1/2
  Demux/1 -> Cos/1, Sin/1, " Body to LPI"/1(phi)  "roll angle"
  Product/1 -> Add7/1
  Add7/1 -> Divide/1
  Cos/1 -> Product1/1
  " Body Velocity"/1 -> Scope1/1, MatrixMultiply/2
  Demux1/1 -> Terminator/1
  Demux/3 -> Terminator1/1  "yaw angle"
  " Euler Angle "/1 -> Demux/1
  Body Rates/1 -> Demux1/1

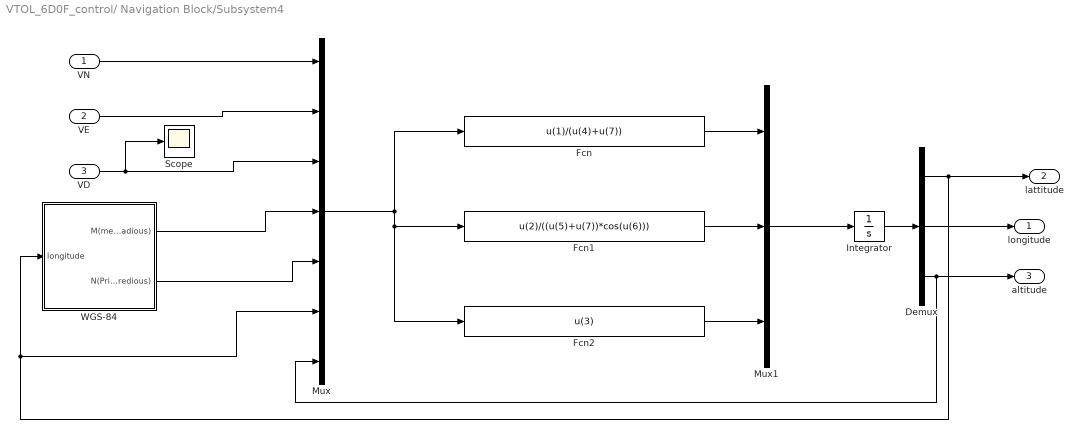
== system VTOL_6D0F_control/ Navigation Block/Subsystem4 ==
  " VN" : Inport
  " VE" : Inport  Port=2
  VD : Inport  Port=3
  " WGS-84" : Subsystem
  Demux : Demux  Outputs=03
  Fcn : Fcn  Expr=u(1)/(u(4)+u(7))
  Fcn1 : Fcn  Expr=u(2)/((u(5)+u(7))*cos(u(6)))
  Fcn2 : Fcn  Expr=u(3)
  Integrator : Integrator
  Mux : Mux  Inputs=07
  Mux1 : Mux  Inputs=03
  Scope : Scope
  longitude : Outport
  " lattitude" : Outport  Port=2
  " altitude" : Outport  Port=3
  wires:
  " VN"/1 -> Mux/1
  " VE"/1 -> Mux/2
  VD/1 -> Scope/1, Mux/3
  " WGS-84"/1(" M(meridian Radious)") -> Mux/4
  " WGS-84"/2(" N(Prime vertical redious)") -> Mux/5
  Demux/1 -> " lattitude"/1, Mux/6, " WGS-84"/1(" longitude")
  Demux/3 -> " altitude"/1, Mux/7
  Mux/1 -> Fcn2/1, Fcn1/1, Fcn/1
  Fcn/1 -> Mux1/1
  Fcn1/1 -> Mux1/2
  Fcn2/1 -> Mux1/3
  Mux1/1 -> Integrator/1
  Integrator/1 -> Demux/1
  Demux/2 -> longitude/1

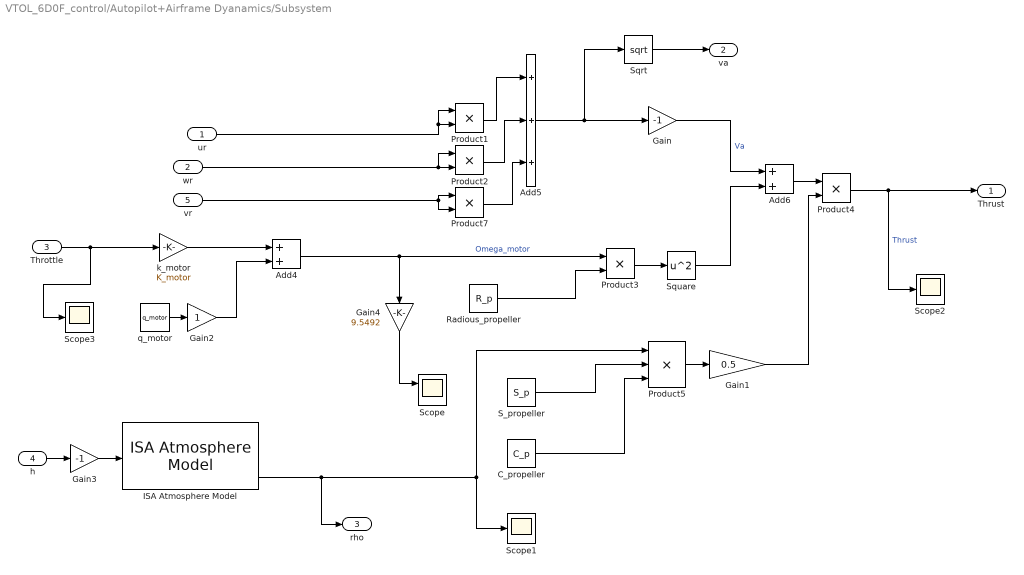
== system VTOL_6D0F_control/Autopilot+Airframe Dyanamics/Subsystem ==
  ur : Inport
  wr : Inport  Port=2
  " Throttle" : Inport  Port=3
  " h" : Inport  Port=4
  " vr" : Inport  Port=5
  " C_propeller" : Constant  Value=C_p
  " Radious_propeller" : Constant  Value=R_p
  " S_propeller" : Constant  Value=S_p
  " k_motor" : Gain  Gain=K_motor
  " q_motor" : Constant  Value=q_motor
  Add4 : Sum
  Add5 : Sum  Inputs=+++
  Add6 : Sum
  Gain : Gain  Gain=-1
  Gain1 : Gain  Gain=0.5
  Gain2 : Gain  Gain=1
  Gain3 : Gain  Gain=-1
  Gain4 : Gain  Gain=9.5492
  ISA Atmosphere Model : aerolibatmos2/ISA Atmosphere Model  custom=off  g=9.80665  gamma=1.4  R=287.0531  L=0.0065  h_trop=11000  h_strat=20000  rho0=1.225  P0=101325  T0=288.15  h0=0
  Product{1..4,7} (5 alike) : Product
  Product5 : Product  Inputs=03
  Scope : Scope  NumInputPorts=2
  Scope1 : Scope
  Scope2 : Scope
  Scope3 : Scope
  Sqrt : Sqrt
  Square : Math  Operator=square
  Thrust : Outport
  " va" : Outport  Port=2
  " rho" : Outport  Port=3
  wires:
  Gain/1 -> Add6/1  "Va"
  Product3/1 -> Square/1
  Gain1/1 -> Product4/2
  " Radious_propeller"/1 -> Product3/2
  ur/1 -> Product1/1, Product1/2
  Product2/1 -> Add5/2
  Product4/1 -> Scope2/1, Thrust/1  "Thrust"
  " Throttle"/1 -> Scope3/1, " k_motor"/1
  Add4/1 -> Product3/1, Gain4/1  "Omega_motor"
  Square/1 -> Add6/2
  " S_propeller"/1 -> Product5/2
  Product1/1 -> Add5/1
  " q_motor"/1 -> Gain2/1
  Add6/1 -> Product4/1
  Product5/1 -> Gain1/1
  " k_motor"/1 -> Add4/1
  Add5/1 -> Sqrt/1, Gain/1
  Gain2/1 -> Add4/2
  " C_propeller"/1 -> Product5/3
  Gain3/1 -> ISA Atmosphere Model/1
  " h"/1 -> Gain3/1
  ISA Atmosphere Model/4 -> " rho"/1, Product5/1, Scope1/1
  wr/1 -> Product2/1, Product2/2
  " vr"/1 -> Product7/1, Product7/2
  Product7/1 -> Add5/3
  Gain4/1 -> Scope/1
  Sqrt/1 -> " va"/1

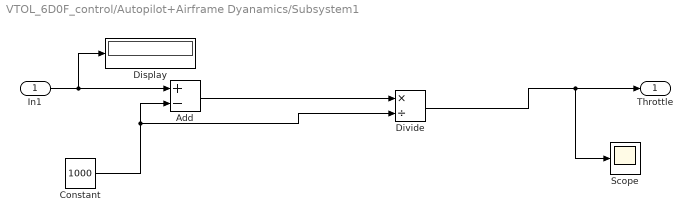
== system VTOL_6D0F_control/Autopilot+Airframe Dyanamics/Subsystem1 ==
  In1 : Inport
  Add : Sum  Inputs=+-
  Constant : Constant  Value=1000
  Display : Display
  Divide : Product  Inputs=*/
  Scope : Scope
  " Throttle" : Outport
  wires:
  In1/1 -> Display/1, Add/1
  Add/1 -> Divide/1
  Constant/1 -> Divide/2, Add/2
  Divide/1 -> Scope/1, " Throttle"/1

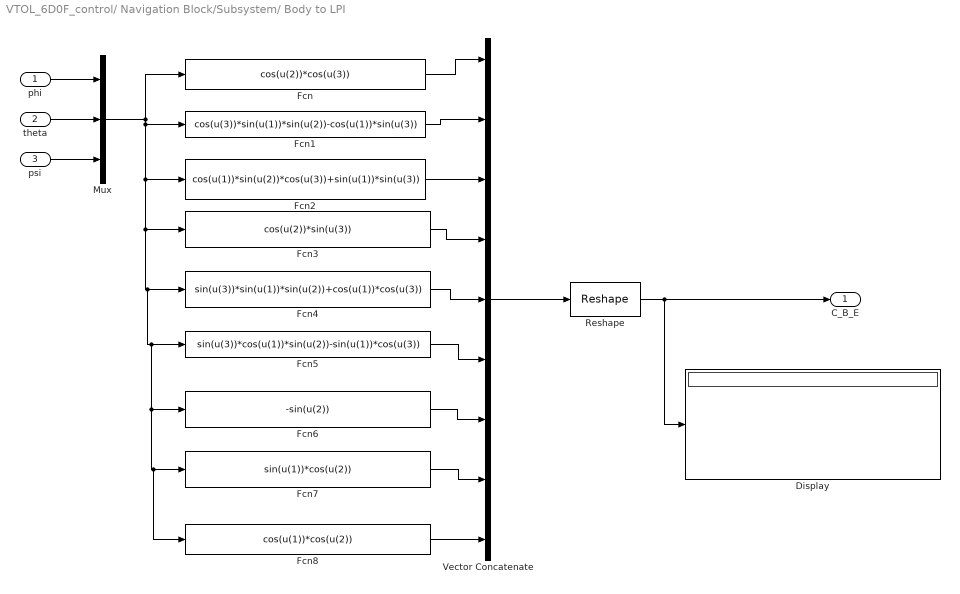
== system VTOL_6D0F_control/ Navigation Block/Subsystem/ Body to LPI ==
  phi : Inport
  theta : Inport  Port=2
  psi : Inport  Port=3
  Display : Display
  Fcn : Fcn  Expr=cos(u(2))*cos(u(3))
  Fcn1 : Fcn  Expr=cos(u(3))*sin(u(1))*sin(u(2))-cos(u(1))*sin(u(3))
  Fcn2 : Fcn  Expr=cos(u(1))*sin(u(2))*cos(u(3))+sin(u(1))*sin(u(3))
  Fcn3 : Fcn  Expr=cos(u(2))*sin(u(3))
  Fcn4 : Fcn  Expr=sin(u(3))*sin(u(1))*sin(u(2))+cos(u(1))*cos(u(3))
  Fcn5 : Fcn  Expr=sin(u(3))*cos(u(1))*sin(u(2))-sin(u(1))*cos(u(3))
  Fcn6 : Fcn  Expr=-sin(u(2))
  Fcn7 : Fcn  Expr=sin(u(1))*cos(u(2))
  Fcn8 : Fcn  Expr=cos(u(1))*cos(u(2))
  Mux : Mux  Inputs=3
  Reshape : Reshape  OutputDimensionality=Customize  OutputDimensions=[3,3]
  Vector Concatenate : Concatenate  NumInputs=09
  C_B_E : Outport
  wires:
  Fcn1/1 -> Vector Concatenate/2
  Fcn4/1 -> Vector Concatenate/5
  Mux/1 -> Fcn8/1, Fcn7/1, Fcn6/1, Fcn5/1, Fcn4/1, Fcn3/1, Fcn2/1, Fcn1/1, Fcn/1
  theta/1 -> Mux/2
  Fcn8/1 -> Vector Concatenate/9
  Fcn6/1 -> Vector Concatenate/7
  Fcn5/1 -> Vector Concatenate/6
  Fcn2/1 -> Vector Concatenate/3
  Fcn/1 -> Vector Concatenate/1
  Fcn3/1 -> Vector Concatenate/4
  Fcn7/1 -> Vector Concatenate/8
  phi/1 -> Mux/1
  psi/1 -> Mux/3
  Vector Concatenate/1 -> Reshape/1
  Reshape/1 -> C_B_E/1, Display/1

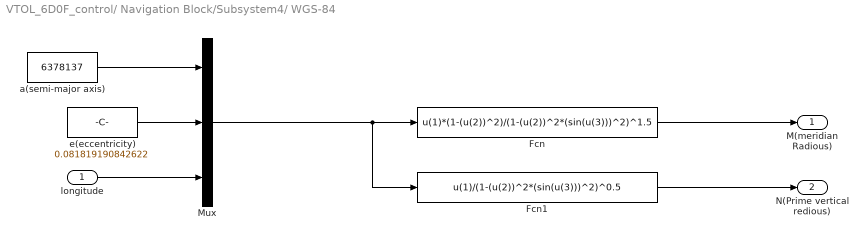
== system VTOL_6D0F_control/ Navigation Block/Subsystem4/ WGS-84 ==
  " longitude" : Inport
  " e(eccentricity)" : Constant  Value=0.081819190842622
  Fcn : Fcn  Expr=u(1)*(1-(u(2))^2)/(1-(u(2))^2*(sin(u(3)))^2)^1.5
  Fcn1 : Fcn  Expr=u(1)/(1-(u(2))^2*(sin(u(3)))^2)^0.5
  Mux : Mux  Inputs=03
  a(semi-major axis) : Constant  Value=6378137
  " M(meridian Radious)" : Outport
  " N(Prime vertical redious)" : Outport  Port=2
  wires:
  " e(eccentricity)"/1 -> Mux/2
  a(semi-major axis)/1 -> Mux/1
  " longitude"/1 -> Mux/3
  Mux/1 -> Fcn1/1, Fcn/1
  Fcn/1 -> " M(meridian Radious)"/1
  Fcn1/1 -> " N(Prime vertical redious)"/1

== matlab function VTOL_6D0F_control/Guidance Mode (u,h,heading Command)/MATLAB Function ==
  data: y output; t input
function y = fcn(t)
  y=-1.2*t;
  
 end

== matlab function VTOL_6D0F_control/Guidance Mode (u,h,heading Command)/MATLAB Function3 ==
  data: omega_t output; t input
function omega_t  = fcn(t)

     omega_t=0;
 
end

== matlab function VTOL_6D0F_control/Guidance Mode (u,h,heading Command)/MATLAB Function1 ==
  data: y output; t input
function y = fcn(t)
 if (t<=600)
    y=-t/12;
 elseif(t>600 && t<=1800)
     y=-50;
 elseif(t>=1800 && t<=2400)
     y=t/12-200;
 else
    y=0;
 end
